simulink model "LQI"  (R2025b)
settings: Solver=FixedStepAuto  StartTime=0.0  StopTime=20  FixedStep=0.01  RelTol=1e-3
settings Model: Creator=flyin  LastModifiedBy=flyin

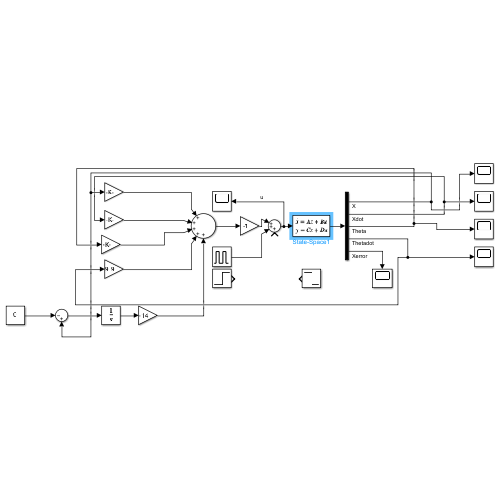
[thumbnail: Simulink's stored preview of the top-level diagram]
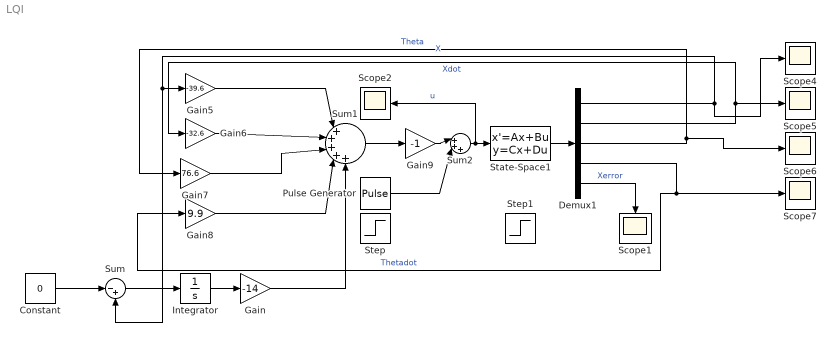
== system LQI ==
  Constant : Constant  Value=0
  Demux1 : Demux  Outputs=5
  Gain : Gain  Gain=-14
  Gain5 : Gain  Gain=-39.6
  Gain6 : Gain  Gain=-32.6
  Gain7 : Gain  Gain=76.6
  Gain8 : Gain  Gain=9.9
  Gain9 : Gain  Gain=-1
  Integrator : Integrator
  Pulse Generator : DiscretePulseGenerator  PulseType=Time based  Amplitude=-6  Period=100  PulseWidth=0.05
  Scope{1..2,4..7} (6 alike) : Scope
      Scope1 settings: ActiveDisplayYMinimum=-0.0075801756397008771  ActiveDisplayYMaximum=0.0014370891550319026
      Scope2 settings: ActiveDisplayYMinimum=-9.98713387542333  ActiveDisplayYMaximum=9.9985704306025927  YLabel=u  DataLoggingVariableName=lqiU  DataLoggingSaveFormat=Array
      Scope4 settings: ActiveDisplayYMinimum=-0.22234283109562034  ActiveDisplayYMaximum=0.21997911362144648  YLabel=meter  DataLoggingVariableName=lqiX  DataLoggingSaveFormat=Array
      Scope5 settings: ActiveDisplayYMinimum=-1  ActiveDisplayYMaximum=1  YLabel=Xdot  DataLoggingVariableName=lqiXdot  DataLoggingSaveFormat=Array
      Scope6 settings: ActiveDisplayYMinimum=-0.022156529166994284  ActiveDisplayYMaximum=0.047599582711792189  YLabel=theta  DataLoggingVariableName=lqiTheta  DataLoggingSaveFormat=Array
      Scope7 settings: ActiveDisplayYMinimum=-1  ActiveDisplayYMaximum=1  DataLoggingVariableName=ScopeData7
  State-Space1 : StateSpace  A=[0, 1.0000, 0, 0, 0; 0, -10.0000, 1.6498, -0.0137, 0; 0, 0, 0, 1.0000, 0; 0, -57.1429, 65.5415, -0.5448, 0; 1.0000, 0, 0, 0, 0]  B=|  C=eye(5)  D=[0.0; 0.0; 0.0; 0.0; 0.0]  InitialCondition=[-0.004891171; -0.051106585; 0.006135923; 0.170442327 ; 0.0]
      | [0
      |  ;   2.0000
      |   ;       0
      |  ;  11.4286; 0]
  Step : Step  Time=0  After=8  SampleTime=0
  Step1 : Step  Time=10  After=-8  SampleTime=0
  Sum : Sum  Inputs=|-+
  Sum1 : Sum  Inputs=|+++++
  Sum2 : Sum  Inputs=|+++
  wires:
  Demux1/3 -> Gain7/1, Scope6/1  "Theta"
  Sum1/1 -> Gain9/1
  Gain6/1 -> Sum1/2
  Gain7/1 -> Sum1/3
  Gain8/1 -> Sum1/4
  Demux1/2 -> Gain6/1, Scope5/1  "Xdot"
  Demux1/1 -> Sum/2, Gain5/1, Scope4/1  "X"
  Gain5/1 -> Sum1/1
  Demux1/4 -> Gain8/1, Scope7/1  "Thetadot"
  Demux1/5 -> Scope1/1  "Xerror"
  Constant/1 -> Sum/1
  Sum/1 -> Integrator/1
  Gain/1 -> Sum1/5
  Integrator/1 -> Gain/1
  State-Space1/1 -> Demux1/1
  Gain9/1 -> Sum2/1
  Sum2/1 -> Scope2/1, State-Space1/1  "u"
  Pulse Generator/1 -> Sum2/2
